simulink model "SimulinkModel_hquad_lin_pitch_kalman_SI"  (Simulink 7.6)
settings: Solver=ode45  StartTime=0.0  StopTime=10.0  RelTol=1e-3
values from neighbouring files (symbols this model uses):
  g = 9.8065    [kostas_malakies.mat]    (also in kostas_malakies2.mat; load_PMModel.m = 9.81; main_last.m; matlab.mat)
  mass = 0.66    [kostas_malakies.mat]    (also in kostas_malakies2.mat; load_PMModel.m = 0.687; main_last.m)
libraries: Hqaud_model_LIB_SI x1
settings Model: Creator=andi  LastModifiedBy=burrimi
settings DebuggingCC: StrictBusMsg=Warning

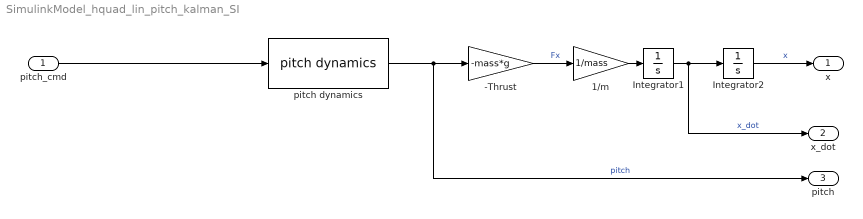
== system SimulinkModel_hquad_lin_pitch_kalman_SI ==
  pitch_cmd : Inport  OutDataTypeStr=double
  -Thrust : Gain  Gain=-mass*g
  1/m : Gain  Gain=1/mass
  Integrator1 : Integrator
  Integrator2 : Integrator
  "pitch dynamics  " : Hqaud_model_LIB_SI/pitch dynamics    SystemSampleTime=-1
  "x  " : Outport
  x_dot : Outport  Port=2
  pitch : Outport  Port=3
  wires:
  pitch_cmd/1 -> "pitch dynamics  "/1
  Integrator2/1 -> "x  "/1  "x"
  1/m/1 -> Integrator1/1
  "pitch dynamics  "/1 -> -Thrust/1, pitch/1  "pitch"
  Integrator1/1 -> Integrator2/1, x_dot/1  "x_dot"
  -Thrust/1 -> 1/m/1  "Fx"
